simulink model "EEL_5661_DC_Motor_sJ_PID_position_110421"  (R2022b)
settings: Solver=VariableStepAuto  StartTime=0.0  StopTime=4  RelTol=1e-3
libraries: simulink x4, slpidlib x1
settings Model: Creator=rothz  LastModifiedBy=Admin
settings SolverCC: AlgebraicLoopSolver=TrustRegion
settings DataIOCC: Refine=5
settings DebuggingCC: UnconnectedInputMsg=warning  UnconnectedOutputMsg=warning  UnconnectedLineMsg=warning  SFMachineParentedDataDiag=warning
settings ModelReferenceCC: EnableRefExpFcnMdlSchedulingChecks=on
settings SFSimCC: CustomCodeUndefinedFunction=UseInterfaceOnly

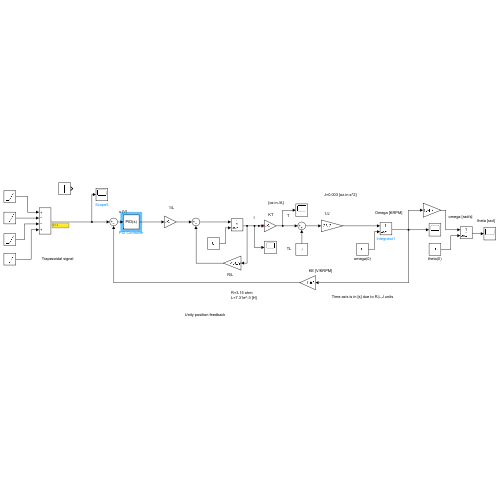
[thumbnail: Simulink's stored preview of the top-level diagram]
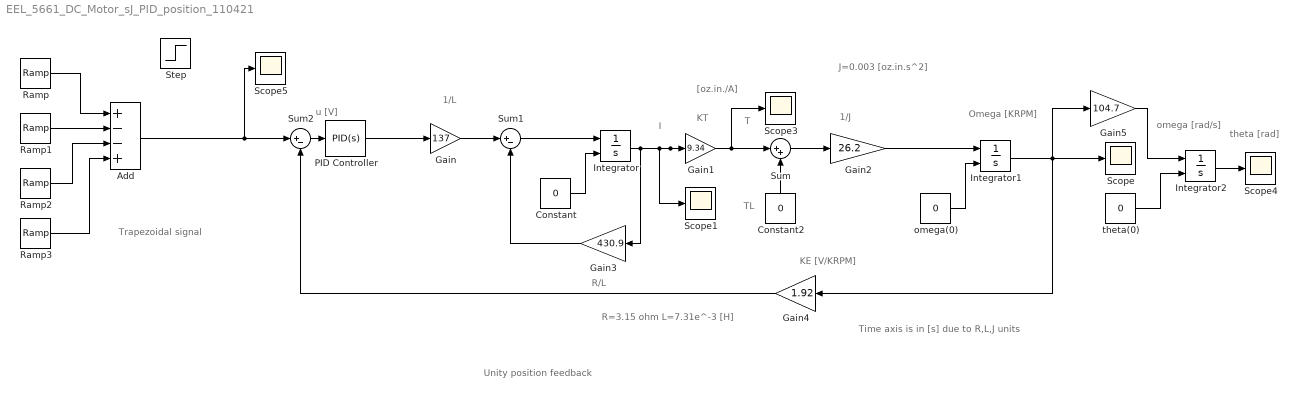
== system EEL_5661_DC_Motor_sJ_PID_position_110421 ==
  note: Trapezoidal signal
  note: Unity position feedback
  note: omega [rad/s]
  note: theta [rad]
  note: Time axis is in [s] due to R,L,J units
  note: R=3.15 ohm
      | L=7.31e^-3 [H]
  note: [oz.in./A]
  note: J=0.003 [oz.in.s^2]
  note: KE [V/KRPM]
  note: u [V]
  note: 1/L
  note: R/L
  note: I
  note: KT
  note: T
  note: TL
  note: 1/J
  note: Omega [KRPM]
  Add : Sum  Inputs=+--+
  Constant : Constant  Value=0
  Constant2 : Constant  Value=0
  Gain : Gain  Gain=137
  Gain1 : Gain  Gain=9.34
  Gain2 : Gain  Gain=26.2
  Gain3 : Gain  Gain=430.9
  Gain4 : Gain  Gain=1.92
  Gain5 : Gain  Gain=104.7
  Integrator : Integrator  InitialConditionSource=external
  Integrator1 : Integrator  InitialConditionSource=external
  Integrator2 : Integrator  InitialConditionSource=external
  PID Controller : slpidlib/PID Controller  Controller=PID  Form=Parallel  TimeDomain=Continuous-time  UseExternalTs=off  SampleTime=-1  IntegratorMethod=Forward Euler  FilterMethod=Forward Euler  ControllerParametersSource=internal  P=1  I=1  UseKiTs=off  D=0  N=100  UseFilter=on  TunerSelectOption=Transfer Function Based (PID Tuner App)  InitialConditionSource=internal  InitialConditionForIntegrator=0  InitialConditionForFilter=0  DifferentiatorICPrevScaledInput=0  ExternalReset=none  TrackingMode=off  Kt=1  LimitOutput=off  SatLimitsSource=internal  UpperSaturationLimit=inf  LowerSaturationLimit=-inf  LinearizeAsGain=on  AntiWindupMode=none  Kb=1  LimitIntegrator=off  UpperIntegratorSaturationLimit=inf  LowerIntegratorSaturationLimit=-inf  POutMin=[]  POutMax=[]  IOutMin=[]  IOutMax=[]  DOutMin=[]  DOutMax=[]  NOutMin=[]  NOutMax=[]  SumOutMin=[]  SumOutMax=[]  SaturationOutMin=[]  SaturationOutMax=[]  PParamMin=[]  PParamMax=[]  IParamMin=[]  IParamMax=[]  DParamMin=[]  DParamMax=[]  NParamMin=[]  NParamMax=[]  KbParamMin=[]  KbParamMax=[]  KtParamMin=[]  KtParamMax=[]  KbOutMin=[]  KbOutMax=[]  KtOutMin=[]  KtOutMax=[]  IntegratorOutMin=[]  IntegratorOutMax=[]  FilterOutMin=[]  FilterOutMax=[]  SumI1OutMin=[]  SumI1OutMax=[]  SumI2OutMin=[]  SumI2OutMax=[]  SumI3OutMin=[]  SumI3OutMax=[]  SumI4OutMin=[]  SumI4OutMax=[]  SumDOutMin=[]  SumDOutMax=[]  DifferentiatorOutMin=[]  DifferentiatorOutMax=[]  FilterDiffOutCoefMin=[]  FilterDiffOutCoefMax=[]  ReciprocalOutMin=[]  ReciprocalOutMax=[]  SumDenOutMin=[]  SumDenOutMax=[]  SumNumOutMin=[]  SumNumOutMax=[]  DivideOutMin=[]  DivideOutMax=[]  UdiffTsProdOutMin=[]  UdiffTsProdOutMax=[]  NTsProdOutMin=[]  NTsProdOutMax=[]  UintegralTsProdOutMin=[]  UintegralTsProdOutMax=[]  UngainTsProdOutMin=[]  UngainTsProdOutMax=[]  ClampingZeroOutDataTypeStr=Inherit: Inherit via back propagation  ClampingZeroOutMin=[]  ClampingZeroOutMax=[]  FilterDenConstantOutDataTypeStr=Inherit: Inherit via back propagation  FilterDenConstantOutMin=[]  FilterDenConstantOutMax=[]  PCopyOutDataTypeStr=Inherit: Inherit via back propagation  PCopyOutMin=[]  PCopyOutMax=[]  NCopyOutDataTypeStr=Inherit: Inherit via back propagation  NCopyOutMin=[]  NCopyOutMax=[]  IntegratorContinuousStateAttributes=''  IntegratorStateMustResolveToSignalObject=off  IntegratorRTWStateStorageClass=Auto  FilterContinuousStateAttributes=''  FilterStateMustResolveToSignalObject=off  FilterRTWStateStorageClass=Auto  ParallelPVariant=InternalParameters  IdealPVariant=Disabled  IVariant=InternalParameters  DVariant=InternalParameters  IntegratorVariant=Continuous  SatVariant=Disabled  AWVariant=Passthrough  PCopyVariant=Disabled  TRVariant=Disabled  FdbkBlocksVariant=Forward  IdealPFdbkVariant=Disabled  SatFdbkVariant=Disabled  DerivativeFilterVariant=ContFilter  NVariant=InternalParameters  NCopyVariant=Disabled  FilterICVariant=InternalICsFilter  IntegratorICVariant=InternalICs  ExternalResetVariant=Disabled  TRSumVariant=Passthrough  SumFdbkVariant=Disabled  SumVariant=Sum_PID  TsampFilterVariant=InternalTs  TsampNgainVariant=Passthrough  TsampIntegralVariant=Passthrough  ExternalSaturationOutDataTypeStr=Inherit: Same as second input
  Ramp : simulink/Sources/Ramp  slope=240  start=0.10  InitialOutput=0
  Ramp1 : simulink/Sources/Ramp  slope=183  start=0.05  InitialOutput=0
  Ramp2 : simulink/Sources/Ramp  slope=183  start=0.05  InitialOutput=0
  Ramp3 : simulink/Sources/Ramp  slope=183  start=0.05  InitialOutput=0
  Scope{,1,3..5} (5 alike) : Scope
  Step : Step  Time=10  SampleTime=0
  Sum : Sum  Inputs=|++
  Sum1 : Sum  Inputs=|+-
  Sum2 : Sum  Inputs=|+-
  omega(0) : Constant  Value=0
  theta(0) : Constant  Value=0
  wires:
  Sum2/1 -> PID Controller/1
  Gain/1 -> Sum1/1
  Sum1/1 -> Integrator/1
  Gain3/1 -> Sum1/2
  Integrator/1 -> Gain1/1, Scope1/1, Gain3/1
  Gain1/1 -> Sum/1, Scope3/1
  Gain2/1 -> Integrator1/1
  Sum/1 -> Gain2/1
  omega(0)/1 -> Integrator1/2
  Constant/1 -> Integrator/2
  Constant2/1 -> Sum/2
  Gain4/1 -> Sum2/2
  Gain5/1 -> Integrator2/1
  Integrator2/1 -> Scope4/1
  theta(0)/1 -> Integrator2/2
  Ramp/1 -> Add/1
  Ramp1/1 -> Add/2
  Ramp2/1 -> Add/3
  Ramp3/1 -> Add/4
  Integrator1/1 -> Gain5/1, Gain4/1, Scope/1
  Add/1 -> Scope5/1, Sum2/1
  PID Controller/1 -> Gain/1
